simulink model "TP_Telecom"  (R2020a)
settings: Solver=FixedStepDiscrete  StartTime=0.0  StopTime=12  RelTol=1e-3
libraries: dspsigops x2, commutil2 x2, commrandsrc3 x1
settings Model: Creator=iba  LastModifiedBy=iba

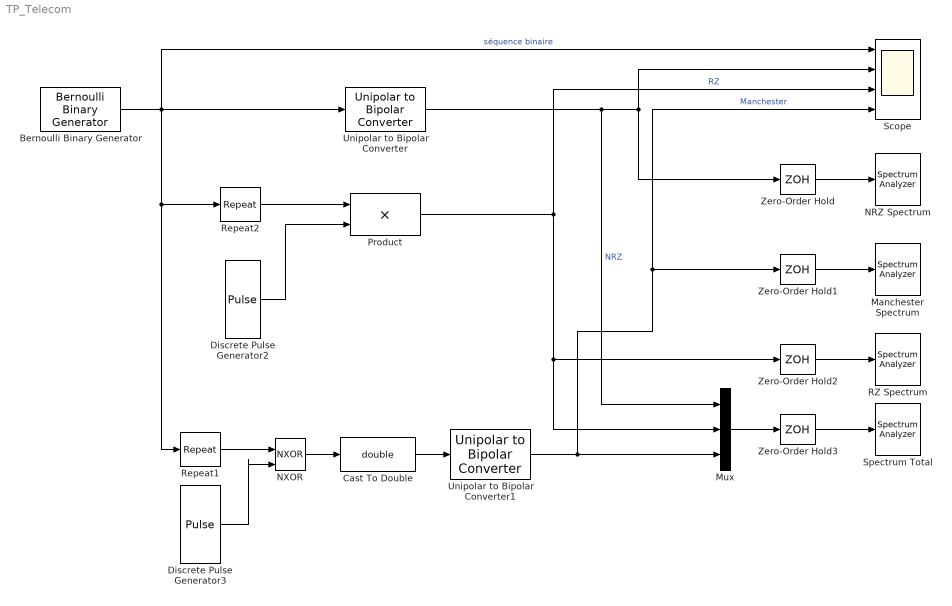
== system TP_Telecom ==
  " NRZ Spectrum" : SpectrumAnalyzer
  Bernoulli Binary Generator : commrandsrc3/Bernoulli Binary Generator  ProbabilityOfZero=0.5  SeedSource=Parameter  Seed=25.  SampleTime=1  SamplesPerFrame=1  OutputDataType=double  SimulateUsing=Interpreted execution
  Cast To Double : DataTypeConversion  OutDataTypeStr=double
  Discrete Pulse Generator2 : DiscretePulseGenerator  SampleTime=0.5
  Discrete Pulse Generator3 : DiscretePulseGenerator  SampleTime=0.5
  "Manchester Spectrum " : SpectrumAnalyzer
  Mux : Mux  Inputs=3
  "NXOR " : Logic  Operator=NXOR  IconShape=distinctive  AllPortsSameDT=off  OutDataTypeStr=boolean
  Product : Product
  RZ Spectrum : SpectrumAnalyzer
  Repeat1 : dspsigops/Repeat  N=2  InputProcessing=Columns as channels (frame based)  RateOptions=Enforce single-rate processing  ic=0  mode=Unused parameter value
  Repeat2 : dspsigops/Repeat  N=2  InputProcessing=Columns as channels (frame based)  RateOptions=Enforce single-rate processing  ic=0  mode=Unused parameter value
  "Scope " : Scope  NumInputPorts=4
  Spectrum Total : SpectrumAnalyzer
  Unipolar to Bipolar Converter : commutil2/Unipolar to Bipolar Converter  M=2  polarity=Positive  dataType=Inherit via internal rule
  Unipolar to Bipolar Converter1 : commutil2/Unipolar to Bipolar Converter  M=2  polarity=Positive  dataType=Inherit via internal rule
  Zero-Order Hold{,1..3} (4 alike) : ZeroOrderHold  SampleTime=0.01
  wires:
  Zero-Order Hold/1 -> " NRZ Spectrum"/1
  Unipolar to Bipolar Converter/1 -> Mux/1, Zero-Order Hold/1, "Scope "/2  "NRZ"
  Zero-Order Hold1/1 -> "Manchester Spectrum "/1
  Zero-Order Hold2/1 -> RZ Spectrum/1
  Bernoulli Binary Generator/1 -> Repeat2/1, Repeat1/1, Unipolar to Bipolar Converter/1, "Scope "/1  "séquence binaire"
  Cast To Double/1 -> Unipolar to Bipolar Converter1/1
  Discrete Pulse Generator3/1 -> "NXOR "/2
  "NXOR "/1 -> Cast To Double/1
  Repeat1/1 -> "NXOR "/1
  Repeat2/1 -> Product/1
  Product/1 -> Zero-Order Hold2/1, Mux/2, "Scope "/3  "RZ"
  Discrete Pulse Generator2/1 -> Product/2
  Unipolar to Bipolar Converter1/1 -> Mux/3, "Scope "/4, Zero-Order Hold1/1  "Manchester"
  Zero-Order Hold3/1 -> Spectrum Total/1
  Mux/1 -> Zero-Order Hold3/1
